simulink library "carnot"  (R2013b)
settings: Solver=ode45  StartTime=0.0  StopTime=10.0  RelTol=1e-3
undefined symbols (not defined in the file or in its folder): A, acol, Ahabit, Awin, Azimuth_Angle, AziWin, B, C, c1, c4, capc, caph, CarnotCallbacks_Density, CarnotCallbacks_Enthalpy, CarnotCallbacks_Enthalpy2Temperature, CarnotCallbacks_Entropy, CarnotCallbacks_Evaporation_Enthalpy, CarnotCallbacks_GlobalMessageLevel, CarnotCallbacks_Grashof, CarnotCallbacks_Heat_Capacity, CarnotCallbacks_Kinematic_Viscosity, CarnotCallbacks_Prandtl, CarnotCallbacks_Saturation_Property, CarnotCallbacks_Saturation_Temperature, CarnotCallbacks_Saturation_Value_Water, CarnotCallbacks_Specific_Volume, CarnotCallbacks_Thermal_Conductivity, CarnotCallbacks_Vapour_Content, CarnotCallbacks_Vapour_Pressure, con, cond, d, Dd, density, dfin, dia, DiameterLastPiece, DPConstant, dpipe, DPLinear, DPQuadratic, emission_out, fluid, FluidMix, FluidType, FPC, frame, g, GeodeticHeight, Gwin, heat_capacity, hgt, HP, Hroom, ID, inlet, K, l, lin, lpipe ... (+29)
undefined symbols (not defined in the file): c2, c3, c5, c6, cwall, dactive, height, mc, mID, rho, tau, UAneighbour, UAwall, uloss
libraries: carnot x333, simulink x25, simulink_extras x7
(part 14 of 16)

== system carnot/Load/Houses/room_nodes/Room_Node ==
  note: r: radiative
      | c: convective
  note: NODE of a ZONE ( heat flow, temperature, ventilation / infiltration and energy consumption)
  sum([S]) : Inport
  1/s to 1/h : Gain  Gain=3600  SaturateOnIntegerOverflow=on  OutDataTypeStr=Inherit: Same as input  ParamDataTypeStr=Inherit: Same as input
  Demux2 : Demux  Outputs=13
  Mux2 : Mux  Inputs=6
  Mux3 : Mux  Inputs=9
  Sensitive room temperature : Subsystem  mask(SENSITIVE TEMPERATURE){share_c=47}
      mask prompts: share_c "SHARE of convective sensitivity, [0,100%]:"
      mask help:
      | This block merges the convective and radiative zone node temperature to the SENSITIVE ZONE TEMPERATURE (weighted arithmetic average of both components).
      |
      | [T] = [Tc; Tr]:  temperature vector of node, °C
      | Ts:              sensitive zone temperature, °C
      mask init: same as carnot/Outputs/Sensitive_Room_Temperature
  Terminator : Terminator
  convective_node : Subsystem
  m^3 : Constant  Value=zoneairvolume
  radiative_node : Subsystem
  "[AIV]" : Outport
  "[S]" : Outport  Port=2
  Qdot_sol : Outport  Port=3
  Vair : Outport  Port=4
  wires:
  m^3/1 -> Vair/1
  Mux2/1 -> Terminator/1  "[Qdot]"
  sum([S])/1 -> "[S]"/1, Demux2/1
  Demux2/8 -> radiative_node/1(Qdotr)  "Qdotr"
  Demux2/7 -> convective_node/1(Qdotc)  "Qdotc"
  Demux2/6 -> Mux2/6  "Qdot_air"
  Demux2/5 -> Mux2/5  "Qdot_heat"
  Demux2/4 -> Mux2/4  "Qdot_pers"
  Demux2/3 -> Mux2/3  "Qdot_light"
  Demux2/2 -> Mux2/2  "Qdot_equip"
  Demux2/1 -> Mux2/1, Qdot_sol/1  "Qdot_sol"
  1/s to 1/h/1 -> Mux3/9  "nair_out"
  convective_node/2(x_H2O) -> Mux3/4  "x_H2O"
  convective_node/3(x_CO2) -> Mux3/5  "x_CO2"
  convective_node/6(p) -> Mux3/8  "p"
  convective_node/5(cp) -> Mux3/7  "cp"
  convective_node/4(rho) -> Mux3/6  "rho"
  convective_node/7(nair_out) -> 1/s to 1/h/1
  convective_node/1(Tc) -> Sensitive room temperature/2(Tc), Mux3/2  "Tc"
  radiative_node/1(Tr) -> Sensitive room temperature/1(Tr), Mux3/3  "Tr"
  Demux2/9 -> convective_node/2(mdot_air)  "mdot_air"
  Demux2/10 -> convective_node/3(mdot_H2O)  "mdot_H2O"
  Demux2/11 -> convective_node/4(mdot_CO2)  "mdot_CO2"
  Demux2/12 -> convective_node/5(Vdot_out2in)  "Vdot_out2in"
  Demux2/13 -> convective_node/6(Vdot_in2out)  "Vdot_in2out"
  Mux3/1 -> "[AIV]"/1
  Sensitive room temperature/1(Ts) -> Mux3/1  "Ts"

== system carnot/Load/Houses/ventilation_heating/Floorheating_TABS ==
  note: source: Koschenz, M.; Lehmann, B.: Thermoaktive Bauteilsysteme tabs. EMPA, Dübendorf, 2000. ISBN 3-905594-19-6
  T(P) : Inport
  THBin : Inport  Port=2
  Bus Assignment : BusAssignment  AssignedSignals=Temperature
  Bus Selector : BusSelector  OutputSignals=Temperature,MassFlow,Pressure,FluidType,FluidMix
  Demux2 : Demux  Outputs=2
  Mux2 : Mux  Inputs=6
  S-Function : S-Function  FunctionName=tabs  Parameters=d d1 d_pipe dr dx l lambda_r lambda_b  EnableBusSupport=off
  power : Outport
  THBout : Outport  Port=2  InitialOutput=0
  wires:
  T(P)/1 -> Mux2/6
  THBin/1 -> Bus Assignment/1, Bus Selector/1
  Bus Selector/4 -> Mux2/4  "<FluidType>"
  Bus Selector/3 -> Mux2/3  "<Pressure>"
  Bus Selector/2 -> Mux2/2  "<MassFlow>"
  Bus Selector/5 -> Mux2/5  "<FluidMix>"
  Bus Selector/1 -> Mux2/1  "<Temperature>"
  Mux2/1 -> S-Function/1
  S-Function/1 -> Demux2/1
  Demux2/2 -> Bus Assignment/2  "Temperature"
  Demux2/1 -> power/1
  Bus Assignment/1 -> THBout/1

== system carnot/Load/Houses/ventilation_heating/THB_P_adapter ==
  note: (°C)
  T(P) : Inport
  THBin : Inport  Port=2
  -1 : Gain  Gain=-1  SaturateOnIntegerOverflow=on  OutDataTypeStr=Inherit: Same as input  ParamDataTypeStr=Inherit: Same as input
  Bus Assignment : BusAssignment  AssignedSignals=Temperature
  Bus Selector : BusSelector  OutputSignals=Temperature,MassFlow
  Heat_Capacity : carnot/Basic/Material_Properties/Heat_Capacity  VariantControl=CarlibClassic  INPUTARGUMENTS=THB  DEBUGLEVEL=DEBUGLEVEL  MAXTOTALWARNINGS=inf  MAXCONSECUTIVEWARNINGS=inf  WRITETOFILE=0  FILENAME='errors.txt'
  Integrator : Integrator  InitialCondition=t0
  Product1 : Product  Inputs=3  SaturateOnIntegerOverflow=on  InputSameDT=on  OutDataTypeStr=Inherit: Same as first input
  Product2 : Product  Inputs=/*  SaturateOnIntegerOverflow=on  InputSameDT=on  OutDataTypeStr=Inherit: Same as first input
  Sum1 : Sum  Inputs=-+  SaturateOnIntegerOverflow=on  InputSameDT=on  OutDataTypeStr=Inherit: Same as first input
  Sum2 : Sum  SaturateOnIntegerOverflow=on  InputSameDT=on  OutDataTypeStr=Inherit: Same as first input
  Sum3 : Sum  Inputs=+-  SaturateOnIntegerOverflow=on  InputSameDT=on  OutDataTypeStr=Inherit: Same as first input
  heat transfer : Gain  Gain=ua  SaturateOnIntegerOverflow=on  OutDataTypeStr=Inherit: Same as input  ParamDataTypeStr=Inherit: Same as input
  mass : Gain  Gain=mass  SaturateOnIntegerOverflow=on  OutDataTypeStr=Inherit: Same as input  ParamDataTypeStr=Inherit: Same as input
  power : Outport  InitialOutput=0
  THB : Outport  Port=2  InitialOutput=0
  wires:
  Bus Assignment/1 -> THB/1
  Sum3/1 -> Product1/1
  Bus Selector/2 -> Product1/2  "<MassFlow>"
  Product1/1 -> Sum2/1
  Heat_Capacity/1 -> Product1/3, mass/1
  Bus Selector/1 -> Sum3/1  "<Temperature>"
  Sum1/1 -> heat transfer/1
  T(P)/1 -> Sum1/2  "Tnode"
  Integrator/1 -> Sum1/1, Bus Assignment/2, Sum3/2  "Twater"
  mass/1 -> Product2/1
  Product2/1 -> Integrator/1
  Sum2/1 -> Product2/2
  -1/1 -> power/1
  heat transfer/1 -> Sum2/2, -1/1  "Qdot"
  THBin/1 -> Heat_Capacity/1, Bus Assignment/1, Bus Selector/1

== system carnot/Load/Houses/wall_floor/Floor_in ==
  "[AIV]floor" : Inport
  power per node : Inport  Port=2
  "[AIV]ceiling" : Inport  Port=3
  Qdot_sol : Inport  Port=4
  Mux : Mux  Inputs=3
  Wall_basic : carnot/Basic/Thermal_Models/Wall_basic  tau=tau  t0=t0  d=d  dactive=dactive  cond=cond  cwall=cwall  rho=rho
  alfa_ceiling : carnot/Load/Houses/heat_transfer/alfa_ceiling  active=active  emission_c=emission_c  wallsurface=wallsurface
  alfa_floor : carnot/Load/Houses/heat_transfer/alfa_floor  active=active  emission_f=emission_f  wallsurface=wallsurface
  per surface : Gain  Gain=1/wallsurface  SaturateOnIntegerOverflow=on  OutDataTypeStr=Inherit: Same as input  ParamDataTypeStr=Inherit: Same as input
  "[S]floor" : Outport
  T(P) : Outport  Port=2
  "[S]ceiling" : Outport  Port=3
  Tn : Outport  Port=4
  wires:
  Wall_basic/2 -> Mux/2, T(P)/1
  "[AIV]ceiling"/1 -> alfa_ceiling/2
  alfa_ceiling/2 -> "[S]ceiling"/1
  alfa_floor/2 -> "[S]floor"/1
  "[AIV]floor"/1 -> alfa_floor/2
  Wall_basic/3 -> Mux/3, alfa_ceiling/1
  Wall_basic/1 -> Mux/1, alfa_floor/1
  alfa_floor/1 -> Wall_basic/1
  alfa_ceiling/1 -> Wall_basic/3
  Qdot_sol/1 -> alfa_floor/3
  power per node/1 -> per surface/1
  per surface/1 -> Wall_basic/2
  Mux/1 -> Tn/1

== system carnot/Load/Houses/wall_floor/Roof ==
  WDB : Inport
  power per node : Inport  Port=2
  "[AIV]" : Inport  Port=3
  Mux : Mux  Inputs=3
  Wall_basic : carnot/Basic/Thermal_Models/Wall_basic  tau=tau  t0=t0  d=d  dactive=dactive  cond=cond  cwall=cwall  rho=rho
  alfa_ceiling : carnot/Load/Houses/heat_transfer/alfa_ceiling  active=active  emission_c=emission_c  wallsurface=wallsurface
  alfa_wall_out : carnot/Load/Houses/heat_transfer/alfa_wall_out  pos=0  absorption_out=0.4  emission_out=0.7  wallsurface=1
  per surface : Gain  Gain=1/wallsurface  SaturateOnIntegerOverflow=on  OutDataTypeStr=Inherit: Same as input  ParamDataTypeStr=Inherit: Same as input
  "[S]" : Outport
  Tn : Outport  Port=2
  wires:
  per surface/1 -> Wall_basic/2
  power per node/1 -> per surface/1
  alfa_ceiling/2 -> "[S]"/1
  "[AIV]"/1 -> alfa_ceiling/2
  alfa_ceiling/1 -> Wall_basic/3
  Wall_basic/2 -> Mux/2
  Wall_basic/3 -> Mux/3, alfa_ceiling/1
  Wall_basic/1 -> Mux/1, alfa_wall_out/2
  WDB/1 -> alfa_wall_out/1
  alfa_wall_out/1 -> Wall_basic/1
  Mux/1 -> Tn/1

== system carnot/Load/Houses/wall_floor/Wall_in ==
  "[AIV]" : Inport
  power per node : Inport  Port=2
  "[AIV]n" : Inport  Port=3
  Mux : Mux  Inputs=3
  Wall_basic : carnot/Basic/Thermal_Models/Wall_basic  tau=tau  t0=t0  d=d  dactive=dactive  cond=cond  cwall=cwall  rho=rho
  alfa_wall_in : carnot/Load/Houses/heat_transfer/alfa_wall_in  active=active  emission_in=emission_in  wallsurface=wallsurface
  alfa_wall_in1 : carnot/Load/Houses/heat_transfer/alfa_wall_in  active=active  emission_in=emission_in  wallsurface=wallsurface
  per surface : Gain  Gain=1/wallsurface  SaturateOnIntegerOverflow=on  OutDataTypeStr=Inherit: Same as input  ParamDataTypeStr=Inherit: Same as input
  "[S]" : Outport
  "[S]n" : Outport  Port=2
  Tn : Outport  Port=3
  wires:
  Mux/1 -> Tn/1
  Wall_basic/2 -> Mux/2
  alfa_wall_in1/2 -> "[S]n"/1
  "[AIV]n"/1 -> alfa_wall_in1/2
  Wall_basic/3 -> alfa_wall_in1/1, Mux/3
  alfa_wall_in1/1 -> Wall_basic/3
  "[AIV]"/1 -> alfa_wall_in/2
  Wall_basic/1 -> Mux/1, alfa_wall_in/1
  alfa_wall_in/2 -> "[S]"/1
  alfa_wall_in/1 -> Wall_basic/1
  per surface/1 -> Wall_basic/2
  power per node/1 -> per surface/1

== system carnot/Load/Houses/wall_floor/Wall_out ==
  WDB : Inport
  power per node : Inport  Port=2
  "[AIV]" : Inport  Port=3
  Mux : Mux  Inputs=3
  Wall_basic : carnot/Basic/Thermal_Models/Wall_basic  tau=tau  t0=t0  d=d  dactive=dactive  cond=cond  cwall=cwall  rho=rho
  alfa_wall_in : carnot/Load/Houses/heat_transfer/alfa_wall_in  active=active  emission_in=emission_in  wallsurface=wallsurface
  alfa_wall_out : carnot/Load/Houses/heat_transfer/alfa_wall_out  pos=pos  absorption_out=absorption_out  emission_out=emission_out  wallsurface=wallsurface
  per surface : Gain  Gain=1/wallsurface  SaturateOnIntegerOverflow=on  OutDataTypeStr=Inherit: Same as input  ParamDataTypeStr=Inherit: Same as input
  "[S]" : Outport
  Tn : Outport  Port=2
  wires:
  alfa_wall_in/2 -> "[S]"/1
  "[AIV]"/1 -> alfa_wall_in/2
  Wall_basic/3 -> Mux/3, alfa_wall_in/1
  alfa_wall_in/1 -> Wall_basic/3
  Wall_basic/1 -> Mux/1, alfa_wall_out/2
  alfa_wall_out/1 -> Wall_basic/1
  per surface/1 -> Wall_basic/2
  power per node/1 -> per surface/1
  WDB/1 -> alfa_wall_out/1
  Wall_basic/2 -> Mux/2
  Mux/1 -> Tn/1

== system carnot/Load/Houses/wall_floor/Wall_with_Window ==
  WDB : Inport
  "[AIV]" : Inport  Port=2
  Ground : Ground
  Wall_out : carnot/Load/Houses/wall_floor/Wall_out  wallsize=[wallsize windowsize]  pos=pos  t0=t0  d=[0.1 0.38]  cond=[0.04 0.79]  cwall=[0.28 0.28]*3600  rho=[900 1800]  reflectground=0.3  abs_emiss=[0.65 0.97 0.96]  tau=tau  dactive=-1
  Window : carnot/Load/Houses/wall_floor/Window  wallsize=windowsize  frame=frame  pos=pos  t0=t0  d=[0.03 0.03]  cond=[.81 .81]  cwall=[.28 .28]*3600  rho=[2500 2500]  misc=[0.2 0.1 1 1]  gvalue=g  tau=tau  dactive=[0.01 0.05]
  "[S]wall" : Outport
  "[S]window" : Outport  Port=2
  wires:
  Window/1 -> "[S]window"/1
  Wall_out/1 -> "[S]wall"/1
  Ground/1 -> Wall_out/2
  "[AIV]"/1 -> Window/2, Wall_out/3
  WDB/1 -> Window/1, Wall_out/1

== system carnot/Load/Houses/wall_floor/Window ==
  WDB : Inport
  "[AIV]" : Inport  Port=2
  Terminator1 : Terminator
  Wall_basic : carnot/Basic/Thermal_Models/Wall_basic  tau=tau  t0=t0  d=d  dactive=dactive  cond=cond  cwall=cwall  rho=rho
  alfa_window_in : carnot/Load/Houses/heat_transfer/alfa_window_in  gvalue=0.7  emission_in=0.87  wallsurface=1  frame=0.1  numlayer=2
  alfa_window_out : carnot/Load/Houses/heat_transfer/alfa_window_out  pos=0  absorption_out=0.01  emission_out=0.87  frame=0.1
  position1 : Constant  Value=gvalue
  "[S]" : Outport
  wires:
  Wall_basic/1 -> alfa_window_out/3
  position1/1 -> alfa_window_out/2
  "[AIV]"/1 -> alfa_window_in/3
  alfa_window_in/1 -> Wall_basic/3
  alfa_window_in/3 -> "[S]"/1
  WDB/1 -> alfa_window_out/1
  alfa_window_out/1 -> alfa_window_in/2
  Wall_basic/2 -> Terminator1/1
  alfa_window_out/2 -> Wall_basic/1
  Wall_basic/3 -> alfa_window_in/1
  alfa_window_in/2 -> Wall_basic/2

== system carnot/Load/Houses/wall_floor/Window_Optics ==
  WDB : Inport
  Bus Selector : BusSelector  OutputSignals=Incidence_Angle_sun,Solar_Radiation_direct_surface,Solar_Radiation_diffuse_surface
  IAM diffuse : Gain  Gain=0.8  SaturateOnIntegerOverflow=on  OutDataTypeStr=Inherit: Same as input  ParamDataTypeStr=Inherit: Same as input
  IAM window : Lookup  InputValues=[-10 0 50 70 80 90]  Table="[1.0 1.0  0.95  0.7  0.0  0.0]"  SaturateOnIntegerOverflow=on
  Product : Product
  Sum : Sum  SaturateOnIntegerOverflow=on  InputSameDT=on  OutDataTypeStr=Inherit: Same as first input
  qsolar : Outport
  wires:
  Bus Selector/3 -> IAM diffuse/1  "<Solar_Radiation_diffuse_surface>"
  IAM window/1 -> Product/1
  IAM diffuse/1 -> Sum/2
  Product/1 -> Sum/1
  Sum/1 -> qsolar/1
  Bus Selector/1 -> IAM window/1  "<Incidence_Angle_sun>"
  Bus Selector/2 -> Product/2  "<Solar_Radiation_direct_surface>"
  WDB/1 -> Bus Selector/1

== system carnot/Load/Houses/wall_floor/Window_with_Shading ==
  WDB : Inport
  "[AIV]" : Inport  Port=2
  control : Inport  Port=3
  alfa_window_in : Subsystem  mask(ALFA){}
      mask help:
      | Convective and radiative heat transfer at the INDOOR SURFACE OF A VERTICAL WINDOW with 1-4 layers (each 3 ... 8 mm thick).
      |
      | Ts  : temperature of window surface, °C,
      | [sun_t]  : sun data (incidence angle, direct and diffuse radiation
      |     at tilted window surface),
      | [AIV]  : conditions of zone node,
      | qdots  : specific heat flow into window construction, W/m^2,
      | [S]  : heat and air flow to zone node.
  alfa_window_out : carnot/Load/Houses/heat_transfer/alfa_window_out  pos=0  absorption_out=0.01  emission_out=0.87  frame=0.1
  lambda_window : Subsystem  mask(LAMBDA){}
      mask help:
      | Heat conduction through a transparent component (window).
      |
      | qdots1	: specific heat flow vertical on surface 1, W/m²
      | qdots2	: specific heat flow vertical on surface 2, W/m²
      | Ts1	: temperature of surface 1, °C
      | Ts2	: temperature of surface 2, °C
      |
      | NOTE CONVENTION for INPUT NUMBER:
      | "1"	  indoor surface of an outer window OR
      | 	  surface "a" of an inner window OR
      |  	  surface "f" of a glass floor
      |
      | "2"	  outdoor surface of a window OR
      | 	  surface "b" of an inner window OR
      |  	  surface "c" of a glass ceiling
  position1 : Constant  Value=gvalue
  "[S]" : Outport
  wires:
  lambda_window/1(Ts1) -> alfa_window_out/3
  WDB/1 -> alfa_window_in/4(WDB), alfa_window_out/1
  "[AIV]"/1 -> alfa_window_in/3("[AIV]")
  alfa_window_in/1(qdots2) -> lambda_window/2(qdots2)
  alfa_window_in/2("[S]") -> "[S]"/1
  lambda_window/2(Ts2) -> alfa_window_in/1(Ts2)
  alfa_window_out/2 -> lambda_window/1(qdots1)
  alfa_window_out/1 -> alfa_window_in/2("[sun_t]")
  control/1 -> alfa_window_in/5(control)
  position1/1 -> alfa_window_out/2

== system carnot/Source/Chiller/Absorption_Chiller_ddT/Transfer Fcn (with initial states) ==
  In1 : Inport
  State Space : StateSpace  A=A  B=B  C=C  D=Dd  X0=X0
  Out1 : Outport  InitialOutput=0
  wires:
  In1/1 -> State Space/1
  State Space/1 -> Out1/1

== system carnot/Source/Chiller/Absorption_Chiller_ddT/absorber // condenser ==
  note: Qdot_E + Qdot_G = Qdot_A + Qdot_C
  THBcooler_in : Inport
  Qdot_E_act [W] : Inport  Port=2
  Qdot_G [W] : Inport  Port=3
  on : Inport  Port=4
  Add1 : Sum
  Bus Assignment : BusAssignment  AssignedSignals=Temperature
  Bus Selector : BusSelector  OutputSignals=Temperature,MassFlow,Pressure,FluidType,FluidMix
  Tcooler_out : Subsystem
  prod : Product
  THBcooler : Outport
  t_AC : Outport  Port=2
  wires:
  Tcooler_out/1(Tcooler_out) -> Bus Assignment/2
  Bus Assignment/1 -> THBcooler/1
  prod/1 -> Tcooler_out/3(Qdot_E + Qdot_G)
  Add1/1 -> prod/2
  on/1 -> prod/1
  Qdot_G [W]/1 -> Add1/2
  Qdot_E_act [W]/1 -> Add1/1
  THBcooler_in/1 -> Bus Assignment/1, Bus Selector/1
  Bus Selector/5 -> Tcooler_out/6(mix)  "<FluidMix>"
  Bus Selector/4 -> Tcooler_out/5(fluid)  "<FluidType>"
  Bus Selector/3 -> Tcooler_out/4(p)  "<Pressure>"
  Bus Selector/1 -> t_AC/1, Tcooler_out/1(T)  "<Temperature>"
  Bus Selector/2 -> Tcooler_out/2(mdot)  "<MassFlow>"

== system carnot/Source/Chiller/Absorption_Chiller_ddT/boiler ==
  THBhot_in : Inport
  deltadelta_t : Inport  Port=2
  on : Inport  Port=3
  Bus Assignment : BusAssignment  AssignedSignals=Temperature
  Bus Selector : BusSelector  OutputSignals=Temperature,MassFlow,Pressure,FluidType,FluidMix
  Pressure_Drop_Fix : carnot/Basic/Pressure_Drop/Pressure_Drop_Fix  con=0  lin=dpg(1)  qua=dpg(2)
  Qdot_G with deltadelta_t : Subsystem
  Thot_out : Subsystem
  prod : Product
  THVhot_out : Outport
  t_B : Outport  Port=2
  Qdot_G [W] : Outport  Port=3
  wires:
  Pressure_Drop_Fix/1 -> THVhot_out/1
  Thot_out/1(Thot_out) -> Bus Assignment/2
  Bus Assignment/1 -> Pressure_Drop_Fix/1
  THBhot_in/1 -> Bus Assignment/1, Bus Selector/1
  Qdot_G with deltadelta_t/1(Qdot_G [W]) -> prod/2
  on/1 -> prod/1
  prod/1 -> Qdot_G [W]/1, Thot_out/3(Qdot_G)
  deltadelta_t/1 -> Qdot_G with deltadelta_t/1(deltadelta_t)
  Bus Selector/5 -> Thot_out/6(mix)  "<FluidMix>"
  Bus Selector/4 -> Thot_out/5(fluid)  "<FluidType>"
  Bus Selector/3 -> Thot_out/4(p)  "<Pressure>"
  Bus Selector/1 -> t_B/1, Thot_out/1(Thot_in)  "<Temperature>"
  Bus Selector/2 -> Thot_out/2(mdot)  "<MassFlow>"

== system carnot/Source/Chiller/Absorption_Chiller_ddT/deltadelta_t ==
  note: deltadelta_t = t_B - (1+E) * t_AC + E * t_E
  t_B : Inport
  t_E : Inport  Port=2
  t_AC : Inport  Port=3
  Add : Sum  Inputs=++-
  Gain : Gain  Gain=1+E
  Gain1 : Gain  Gain=E
  deltadelta_t : Outport
  wires:
  t_AC/1 -> Gain/1
  t_E/1 -> Gain1/1
  Add/1 -> deltadelta_t/1
  t_B/1 -> Add/1
  Gain1/1 -> Add/2
  Gain/1 -> Add/3

== system carnot/Source/Chiller/Absorption_Chiller_ddT/evaporator ==
  THBload_in : Inport
  deltadelta_t : Inport  Port=2
  on : Inport  Port=3
  Bus Assignment : BusAssignment  AssignedSignals=Temperature
  Bus Selector : BusSelector  OutputSignals=Temperature,MassFlow,Pressure,FluidType,FluidMix
  Pressure_Drop_Fix : carnot/Basic/Pressure_Drop/Pressure_Drop_Fix  con=0  lin=dpe(1)  qua=dpe(2)
  Qdot_E with deltadelta_t : Subsystem
  Tchilled_out : Subsystem
  prod : Product
  THBload : Outport
  t_E : Outport  Port=2
  Qdot_E [W] : Outport  Port=3
  wires:
  Pressure_Drop_Fix/1 -> THBload/1
  Bus Assignment/1 -> Pressure_Drop_Fix/1
  THBload_in/1 -> Bus Assignment/1, Bus Selector/1
  Qdot_E with deltadelta_t/1(Qdot_E [W]) -> prod/2
  prod/1 -> Qdot_E [W]/1, Tchilled_out/3(Qdot_E)
  on/1 -> prod/1
  Bus Selector/3 -> Tchilled_out/4(p)  "<Pressure>"
  Tchilled_out/1(Tcold) -> Bus Assignment/2, t_E/1
  deltadelta_t/1 -> Qdot_E with deltadelta_t/1(deltadelta_t)
  Bus Selector/5 -> Tchilled_out/6(mix)  "<FluidMix>"
  Bus Selector/4 -> Tchilled_out/5(fluid)  "<FluidType>"
  Bus Selector/1 -> Tchilled_out/1(T)  "<Temperature>"
  Bus Selector/2 -> Tchilled_out/2(mdot)  "<MassFlow>"

== system carnot/Source/Chiller/Compression_Air_Water_Chiller/Lookup_tables _COP + Q_cold_faktor ==
  T_AIR_IN : Inport
  T_WATER_OUT : Inport  Port=2
  control_AC : Inport  Port=3
  Constant : Constant  Value=Q_Nom
  Gain : Gain  Gain=1000
  Product : Product  RndMeth=Zero
  Product1 : Product  Inputs=4  RndMeth=Zero
  Product2 : Product  Inputs=/*  RndMeth=Zero
  lookup_table_COP : Lookup_n-D  BreakpointsForDimension1=[7,18]  BreakpointsForDimension2=[15,20,25,30,35,40]  BreakpointsForDimension3=[1:2]  BreakpointsForDimension4=[1:2]  Table=[3.55 3.15 2.65 2.25 2 1.7;3.8 3.4 2.93 2.58 2.2 1.95]  InputSameDT=on
  lookup_table_Q_cold_faktor : Lookup_n-D  BreakpointsForDimension1=[7,18]  BreakpointsForDimension2=[15,20,25,30,35,40]  BreakpointsForDimension3=[1:2]  BreakpointsForDimension4=[1:2]  Table=|  InputSameDT=on
      | [ 1.26 1.19 1.08 1.00 0.90 0.79;
      |              1.65 1.53 1.41 1.28 1.18 1.09]
  runtime_AC : Subsystem  TreatAsAtomicUnit=on
      mask help: This block counts the time if input is set to one, it stops counting if input is zero and continues when input rises to one again.
      mask Help: eval('filetest (''manual.htm#count_working_time'')')
  start-up-faktor : Fcn  Expr=1-exp(-u/(150/5))
  COP : Outport
  Q_cold : Outport  Port=2
  P_el : Outport  Port=3
  wires:
  Gain/1 -> Q_cold/1, Product2/2
  T_WATER_OUT/1 -> lookup_table_Q_cold_faktor/1, lookup_table_COP/1
  T_AIR_IN/1 -> lookup_table_Q_cold_faktor/2, lookup_table_COP/2
  lookup_table_COP/1 -> Product/1, Product2/1
  control_AC/1 -> Product/2, runtime_AC/1(control_AC), Product1/2
  lookup_table_Q_cold_faktor/1 -> Product1/3
  runtime_AC/1(runtime) -> start-up-faktor/1
  Product/1 -> COP/1
  Product1/1 -> Gain/1
  start-up-faktor/1 -> Product1/1
  Constant/1 -> Product1/4
  Product2/1 -> P_el/1

== system carnot/Source/Chiller/Compression_Air_Water_Chiller/cooling ==
  THB_in : Inport
  Q_cold : Inport  Port=2
  Bus Assignment : BusAssignment  AssignedSignals=Temperature
  Bus Selector : BusSelector  OutputSignals=Temperature,MassFlow
  Constant : Constant  Value=20
  Constant_THB : carnot/Source/Simple/Constant_THB  t=40  mdot=0*100/3600  p=1e5  mID=No Pressure Drop  fluid=Water  mix=0  dia=0.02  hgt=0
  Heat_Capacity : carnot/Basic/Material_Properties/Heat_Capacity  VariantControl=CarlibClassic  INPUTARGUMENTS=THB  DEBUGLEVEL=DEBUGLEVEL  MAXTOTALWARNINGS=inf  MAXCONSECUTIVEWARNINGS=inf  WRITETOFILE=0  FILENAME='errors.txt'
  Product : Product  Inputs=//*  SaturateOnIntegerOverflow=on  RndMeth=Zero  InputSameDT=on  OutDataTypeStr=Inherit: Same as first input
  Saturation : Saturate  UpperLimit=inf  LowerLimit=1
  Storage_Type_1 : carnot/Storage/Thermal/Storage_Type_1  uloss=1  ubot=1  utop=1  cond=1  t0=[10:5:55]  volume=0.03  dia=0.01  pos=standing cylinder  nconnect=2  nodes=10  mpoints=10
  Sum2 : Sum  Inputs=+-  InputSameDT=on  OutDataTypeStr=Inherit: Same as first input
  Terminator : Terminator
  Terminator1 : Terminator
  Terminator2 : Terminator
  isinf : MATLAB Function  TreatAsAtomicUnit=on
  isnan : MATLAB Function  TreatAsAtomicUnit=on
  THB_out : Outport
  wires:
  Storage_Type_1/3 -> Terminator2/1
  Storage_Type_1/2 -> Terminator1/1
  Storage_Type_1/1 -> Terminator/1
  Storage_Type_1/4 -> THB_out/1
  Bus Selector/2 -> Product/1  "<MassFlow>"
  Heat_Capacity/1 -> Product/2
  Bus Assignment/1 -> Storage_Type_1/3
  Constant/1 -> Storage_Type_1/1
  Constant_THB/1 -> Storage_Type_1/2
  THB_in/1 -> Heat_Capacity/1, Bus Selector/1, Bus Assignment/1
  Bus Selector/1 -> Sum2/1  "<Temperature>"
  Q_cold/1 -> Product/3  "W"
  isnan/1(y) -> isinf/1(u)
  Product/1 -> isnan/1(u)
  isinf/1(y) -> Sum2/2
  Sum2/1 -> Saturation/1
  Saturation/1 -> Bus Assignment/2

== system carnot/Source/Chiller/Compression_Air_Water_Chiller/measure_T_WATER_OUT ==
  THV_in : Inport
  Demux3 : Demux  Outputs=2
  Terminator : Terminator
  heat capacity : StateSpace  A=-tc  B=tc  D=0  X0=t0
  select temperature : Selector  InputPortWidth=5  IndexOptions=Index vector (dialog)  Indices=[2]  OutputSizes=1
  T : Outport
  THV : Outport  Port=2
  wires:
  Demux3/2 -> Terminator/1
  Demux3/1 -> select temperature/1
  THV_in/1 -> Demux3/1, THV/1
  select temperature/1 -> heat capacity/1
  heat capacity/1 -> T/1

== system carnot/Source/Chiller/Cooling_Tower/Fan ==
  note: Grundlage zur Berechnung
      | bei Drehzahländerung eines bestimmten Lüfters
      |
      | Proportionalitätsgesetz
      | V1/V2 = n1/n2
      | P1/P2 = (n1/n2)^3
      |
      | Wirkungsgrad Elektromotor
      | P = Pm/eta
  n_fan : Inport
  Divide1 : Product  Inputs=*/
  Divide2 : Product  Inputs=*/*
  Divide3 : Product  Inputs=/*
  Divide4 : Product  Inputs=/*
  Input Leistung : Constant  Value=1.8
  Math Function : Math  Operator=pow  SaturateOnIntegerOverflow=on
  Pw1 : Constant  Value=3
  max. Drehzahl : Constant  Value=824
  max. Vdot_Lüfter : Constant  Value=2.2
  n_fan [%] : Outport
  vdot_fan : Outport  Port=2
  P_fan : Outport  Port=3
  wires:
  n_fan/1 -> Divide2/1, Divide4/1, Divide1/1
  max. Drehzahl/1 -> Divide2/2, Divide1/2, Divide4/2
  Divide1/1 -> n_fan [%]/1
  Input Leistung/1 -> Divide3/2
  max. Vdot_Lüfter/1 -> Divide2/3
  Divide2/1 -> vdot_fan/1
  Divide3/1 -> P_fan/1
  Divide4/1 -> Math Function/1
  Math Function/1 -> Divide3/1
  Pw1/1 -> Math Function/2

== system carnot/Source/Chiller/Cooling_Tower/Feuchtkugel- temperatureinfluss // wet-bulb temperature effect ==
  WDB : Inport
  t_ie : Inport  Port=2
  Enable : EnablePort
  "Abgleich " : Subsystem
  Add : Sum
  Constant : Constant  Value=2
  Divide : Product  Inputs=*/
  THB_WetBulbTemperature : carnot/Basic/Material_Properties/THB_WetBulbTemperature
  Terminator1 : Terminator
  WDB2THB : carnot/Weather/WDB2THB  dia=0.2
  wet-bulb 15 °C : Subsystem
  t_FK : Outport  InitialOutput=0
  t_ia_FK : Outport  Port=2  InitialOutput=0
  dt : Outport  Port=3  InitialOutput=0
  wires:
  WDB2THB/1 -> THB_WetBulbTemperature/1
  THB_WetBulbTemperature/2 -> Terminator1/1
  WDB/1 -> WDB2THB/1
  wet-bulb 15 °C/1(t_ia_FK15) -> "Abgleich "/3(t_ia_FK15)
  THB_WetBulbTemperature/1 -> "Abgleich "/1(t_FK), t_FK/1
  t_ie/1 -> Add/2, wet-bulb 15 °C/1(t_ie), "Abgleich "/2(t_ie)
  "Abgleich "/1(t_ia_FK) -> Add/1, t_ia_FK/1
  Add/1 -> Divide/1
  Constant/1 -> Divide/2
  Divide/1 -> dt/1

== system carnot/Source/Chiller/Cooling_Tower/Leistungseinflüsse // influence on coolingpower ==
  t_ia_FK : Inport
  cp_i : Inport  Port=2
  t_ie : Inport  Port=3
  mdot_i : Inport  Port=4
  Fluid_Type : Inport  Port=5
  Fluid_mix : Inport  Port=6
  n_fan [%] : Inport  Port=7
  Enable : EnablePort
  Qdot_i_FK : Subsystem
  "Qdot_i_ist " : Subsystem
  "t_ia_ist " : Subsystem
  Qdot_i_ist : Outport  InitialOutput=0
  t_ia_ist : Outport  Port=2  InitialOutput=0
  wires:
  "Qdot_i_ist "/1(Qdot_i_ist) -> Qdot_i_ist/1, "t_ia_ist "/1(Qdot_i_ist)
  Qdot_i_FK/1(Qdot_i_FK) -> "Qdot_i_ist "/1(Qdot_i_FK)
  t_ie/1 -> Qdot_i_FK/2(t_ie), "t_ia_ist "/2(t_ie), "Qdot_i_ist "/6(t_ie)
  t_ia_FK/1 -> Qdot_i_FK/1(t_ia_FK)
  n_fan [%]/1 -> "Qdot_i_ist "/2(n_Fan [%])
  "t_ia_ist "/1(t_ia_ist) -> t_ia_ist/1
  cp_i/1 -> "t_ia_ist "/3(cp_i)
  Fluid_Type/1 -> Qdot_i_FK/3(Fluid_Type), "Qdot_i_ist "/5(Fluid_Type)
  mdot_i/1 -> "Qdot_i_ist "/4(mdot_i), "t_ia_ist "/4(mdot)
  Fluid_mix/1 -> "Qdot_i_ist "/3(Fluid_mix)

== system carnot/Source/Chiller/Cooling_Tower/Verbrauch // consumption ==
  Qdot : Inport
  vdot_fan : Inport  Port=2
  P_fan : Inport  Port=3
  control_fan : Inport  Port=4
  phi_le : Inport  Port=5
  t_le : Inport  Port=6
  t_ie : Inport  Port=7
  Strom : Subsystem
  Verdunstung : Subsystem
  energy : Outport
  power : Outport  Port=2
  Wasserverbrauch : Outport  Port=3
  wires:
  control_fan/1 -> Strom/1(control_Fan), Verdunstung/1(control_Fan)
  P_fan/1 -> Strom/2(P_Fan)
  Strom/2(power) -> power/1
  t_le/1 -> Verdunstung/2(t_le)
  Verdunstung/1(Wasserverbrauch) -> Wasserverbrauch/1
  phi_le/1 -> Verdunstung/3(phi_le)
  vdot_fan/1 -> Verdunstung/4(Vdot_Fan)
  Qdot/1 -> Verdunstung/5(Qdot)
  t_ie/1 -> Verdunstung/6(t_ie)
  Strom/1(energy) -> energy/1

== system carnot/Source/Heat_Exchanger/Radiator_AIV/Troom ==
  "[AIV]" : Inport
  Sum4 : Sum  Inputs=1  SaturateOnIntegerOverflow=on  InputSameDT=on  OutDataTypeStr=Inherit: Same as first input
  gain : Gain  Gain=0.5  SaturateOnIntegerOverflow=on  OutDataTypeStr=Inherit: Same as input  ParamDataTypeStr=Inherit: Same as input
  select Tc Tr : Selector  InputPortWidth=9  IndexOptions=Index vector (dialog)  Indices=[2 3]  OutputSizes=1
  Troom : Outport
  wires:
  select Tc Tr/1 -> Sum4/1
  Sum4/1 -> gain/1
  gain/1 -> Troom/1  "Troom"
  "[AIV]"/1 -> select Tc Tr/1

== system carnot/Source/Heat_Pump/Ground_Source_Heat_Exchanger/Randbedingung 1 ==
  note: Qtot,i
  note: Qup,i
  note: Qdown,i
  T_Up : Inport
  T_Down : Inport  Port=2
  T_Earth(i,1) : Inport  Port=3
  Gain1 : Gain  Gain=L1/(2)  SaturateOnIntegerOverflow=on  OutDataTypeStr=Inherit: Same as input  ParamDataTypeStr=Inherit: Same as input
  Gain2 : Gain  Gain=L1/(2)  SaturateOnIntegerOverflow=on  OutDataTypeStr=Inherit: Same as input  ParamDataTypeStr=Inherit: Same as input
  Gain3 : Gain  Gain=(1)/L1  SaturateOnIntegerOverflow=on  OutDataTypeStr=Inherit: Same as input  ParamDataTypeStr=Inherit: Same as input
  Sum3 : Sum  Inputs=|-+  SaturateOnIntegerOverflow=on  InputSameDT=on  OutDataTypeStr=Inherit: Same as first input
  Sum4 : Sum  Inputs=-+  SaturateOnIntegerOverflow=on  InputSameDT=on  OutDataTypeStr=Inherit: Same as first input
  Sum5 : Sum  Inputs=|++  SaturateOnIntegerOverflow=on  InputSameDT=on  OutDataTypeStr=Inherit: Same as first input
  Sum6 : Sum  Inputs=|-+  SaturateOnIntegerOverflow=on  InputSameDT=on  OutDataTypeStr=Inherit: Same as first input
  T_Earth(i,0) : Outport
  wires:
  Sum6/1 -> T_Earth(i,0)/1
  T_Earth(i,1)/1 -> Sum6/2, Sum4/2, Sum3/2
  T_Up/1 -> Sum4/1
  T_Down/1 -> Sum3/1
  Gain3/1 -> Sum6/1
  Sum5/1 -> Gain3/1
  Gain2/1 -> Sum5/2
  Gain1/1 -> Sum5/1
  Sum4/1 -> Gain2/1
  Sum3/1 -> Gain1/1

== system carnot/Source/Heat_Pump/Ground_Source_Heat_Exchanger/Randbedingung 2 ==
  note: DeltaT
  note: T_Earth(i,DimRad)
  T_Earth(i,0) : Inport
  T_Earth(i,1) : Inport  Port=2
  Dd6 : Gain  Gain=c4  Multiplication=Matrix(K*u)  SaturateOnIntegerOverflow=on  OutDataTypeStr=Inherit: Same as input  ParamDataTypeStr=Inherit: Same as input
  Sum2 : Sum  Inputs=|+-  SaturateOnIntegerOverflow=on  InputSameDT=on  OutDataTypeStr=Inherit: Same as first input
  Sum3 : Sum  Inputs=+-  SaturateOnIntegerOverflow=on  InputSameDT=on  OutDataTypeStr=Inherit: Same as first input
  Tearth DimRad : Constant  Value=T_null  VectorParams1D=off
  g-function : Subsystem
  T_Earth(i,DimRad) Gew : Outport
  T_Earth(i,DimRad) : Outport  Port=2
  wires:
  g-function/1(DeltaT) -> Sum2/2
  Sum3/1 -> g-function/1(T(i,1)-T(i,0))
  Dd6/1 -> T_Earth(i,DimRad) Gew/1
  T_Earth(i,0)/1 -> Sum3/2
  T_Earth(i,1)/1 -> Sum3/1
  Tearth DimRad/1 -> Sum2/1
  Sum2/1 -> T_Earth(i,DimRad)/1, Dd6/1

== system carnot/Source/Heat_Pump/Ground_Source_Heat_Exchanger/Tdown ==
  In1 : Inport
  A mult : Product  Multiplication=Matrix(*)  RndMeth=Zero
  B mult : Product  Multiplication=Matrix(*)  RndMeth=Zero
  C mult : Product  Multiplication=Matrix(*)  RndMeth=Zero
  D mult : Product  Multiplication=Matrix(*)  RndMeth=Zero
  Integrator : Integrator  InitialCondition=Tdown_0
  Selector1 : Selector  InputPortWidth=DimAxi/2  IndexOptions=Index vector (dialog)  Indices=1  OutputSizes=1
  Selector2 : Selector  InputPortWidth=DimAxi/2  IndexOptions=Index vector (dialog)  Indices=2  OutputSizes=1
  Sum1 : Sum  Inputs=|++
  Sum2 : Sum  Inputs=++|
  Out1 : Outport
  Out2 : Outport  Port=2
  Out3 : Outport  Port=3
  wires:
  Sum2/1 -> Selector2/1, Selector1/1, Out1/1  "y"
  In1/1 -> B mult/2, D mult/2
  D mult/1 -> Sum2/1
  C mult/1 -> Sum2/2
  B mult/1 -> Sum1/1
  Sum1/1 -> Integrator/1  "Xdot"
  Integrator/1 -> A mult/2, C mult/2  "X"
  A mult/1 -> Sum1/2
  [B] -> B mult/1
  [A] -> A mult/1
  [C] -> C mult/1
  [D] -> D mult/1
  Selector1/1 -> Out2/1
  Selector2/1 -> Out3/1

== system carnot/Source/Heat_Pump/Ground_Source_Heat_Exchanger/Tup ==
  In1 : Inport
  A mult : Product  Multiplication=Matrix(*)  RndMeth=Zero
  B mult : Product  Multiplication=Matrix(*)  RndMeth=Zero
  C mult : Product  Multiplication=Matrix(*)  RndMeth=Zero
  D mult : Product  Multiplication=Matrix(*)  RndMeth=Zero
  Integrator : Integrator  InitialCondition=Tup_0
  Selector1 : Selector  InputPortWidth=DimAxi/2  IndexOptions=Index vector (dialog)  Indices=1  OutputSizes=1
  Selector2 : Selector  InputPortWidth=DimAxi/2  IndexOptions=Index vector (dialog)  Indices=2  OutputSizes=1
  Sum1 : Sum  Inputs=|++
  Sum2 : Sum  Inputs=++|
  Out1 : Outport
  Out2 : Outport  Port=2
  Out3 : Outport  Port=3
  wires:
  Sum2/1 -> Selector2/1, Selector1/1, Out1/1  "y"
  In1/1 -> B mult/2, D mult/2
  D mult/1 -> Sum2/1
  C mult/1 -> Sum2/2
  B mult/1 -> Sum1/1
  Sum1/1 -> Integrator/1  "Xdot"
  Integrator/1 -> A mult/2, C mult/2  "X"
  A mult/1 -> Sum1/2
  [Bu] -> B mult/1
  [Au] -> A mult/1
  [Cu] -> C mult/1
  [Du] -> D mult/1
  Selector1/1 -> Out2/1
  Selector2/1 -> Out3/1

== system carnot/Source/Heat_Pump/Ground_Source_Heat_Exchanger/mdot>0 ==
  In1 : Inport
  mdot : Inport  Port=2
  In4 : Inport  Port=3
  Add : Sum
  Fcn2 : Fcn  Expr=u>0
  Fcn3 : Fcn  Expr=u==0
  Product : Product  RndMeth=Zero
  Product1 : Product  RndMeth=Zero
  Out1 : Outport
  wires:
  Product/1 -> Add/1
  Product1/1 -> Add/2
  In1/1 -> Product/1
  Add/1 -> Out1/1
  In4/1 -> Product1/2
  mdot/1 -> Fcn2/1, Fcn3/1
  Fcn2/1 -> Product/2
  Fcn3/1 -> Product1/1

== system carnot/Source/Heat_Pump/Ground_Source_Heat_Exchanger/mdot>1 ==
  In1 : Inport
  mdot : Inport  Port=2
  In4 : Inport  Port=3
  Add : Sum
  Fcn2 : Fcn  Expr=u>0
  Fcn3 : Fcn  Expr=u==0
  Product : Product  RndMeth=Zero
  Product1 : Product  RndMeth=Zero
  Out1 : Outport
  wires:
  Product/1 -> Add/1
  Product1/1 -> Add/2
  In1/1 -> Product/1
  Add/1 -> Out1/1
  In4/1 -> Product1/2
  mdot/1 -> Fcn2/1, Fcn3/1
  Fcn2/1 -> Product/2
  Fcn3/1 -> Product1/1

== system carnot/Source/Heat_Pump/Ground_Source_Heat_Exchanger/mdot>2 ==
  In1 : Inport
  mdot : Inport  Port=2
  In4 : Inport  Port=3
  Add : Sum
  Fcn2 : Fcn  Expr=u>0
  Fcn3 : Fcn  Expr=u==0
  Product : Product  RndMeth=Zero
  Product1 : Product  RndMeth=Zero
  Out1 : Outport
  wires:
  Product/1 -> Add/1
  Product1/1 -> Add/2
  In1/1 -> Product/1
  Add/1 -> Out1/1
  In4/1 -> Product1/2
  mdot/1 -> Fcn2/1, Fcn3/1
  Fcn2/1 -> Product/2
  Fcn3/1 -> Product1/1

== system carnot/Source/Heat_Pump/Ground_Source_Heat_Exchanger/mdot>3 ==
  In1 : Inport
  mdot : Inport  Port=2
  In4 : Inport  Port=3
  Add : Sum
  Fcn2 : Fcn  Expr=u>0
  Fcn3 : Fcn  Expr=u==0
  Product : Product  RndMeth=Zero
  Product1 : Product  RndMeth=Zero
  Out1 : Outport
  wires:
  Product/1 -> Add/1
  Product1/1 -> Add/2
  In1/1 -> Product/1
  Add/1 -> Out1/1
  In4/1 -> Product1/2
  mdot/1 -> Fcn2/1, Fcn3/1
  Fcn2/1 -> Product/2
  Fcn3/1 -> Product1/1

== system carnot/Source/Heat_Pump/Ground_Source_Heat_Exchanger/mdot>4 ==
  In1 : Inport
  mdot : Inport  Port=2
  In4 : Inport  Port=3
  Add : Sum
  Fcn2 : Fcn  Expr=u>0
  Fcn3 : Fcn  Expr=u==0
  Product : Product  RndMeth=Zero
  Product1 : Product  RndMeth=Zero
  Out1 : Outport
  wires:
  Product/1 -> Add/1
  Product1/1 -> Add/2
  In1/1 -> Product/1
  Add/1 -> Out1/1
  In4/1 -> Product1/2
  mdot/1 -> Fcn2/1, Fcn3/1
  Fcn2/1 -> Product/2
  Fcn3/1 -> Product1/1

== system carnot/Source/Heat_Pump/Ground_Source_Heat_Exchanger/mdot>5 ==
  In1 : Inport
  mdot : Inport  Port=2
  In4 : Inport  Port=3
  Add : Sum
  Fcn2 : Fcn  Expr=u>0
  Fcn3 : Fcn  Expr=u==0
  Product : Product  RndMeth=Zero
  Product1 : Product  RndMeth=Zero
  Out1 : Outport
  wires:
  Product/1 -> Add/1
  Product1/1 -> Add/2
  In1/1 -> Product/1
  Add/1 -> Out1/1
  In4/1 -> Product1/2
  mdot/1 -> Fcn2/1, Fcn3/1
  Fcn2/1 -> Product/2
  Fcn3/1 -> Product1/1

== system carnot/Source/Heat_Pump/Ground_Source_Heat_Exchanger/mdot>6 ==
  In1 : Inport
  mdot : Inport  Port=2
  In4 : Inport  Port=3
  Add : Sum
  Fcn2 : Fcn  Expr=u>0
  Fcn3 : Fcn  Expr=u==0
  Product : Product  RndMeth=Zero
  Product1 : Product  RndMeth=Zero
  Out1 : Outport
  wires:
  Product/1 -> Add/1
  Product1/1 -> Add/2
  In1/1 -> Product/1
  Add/1 -> Out1/1
  In4/1 -> Product1/2
  mdot/1 -> Fcn2/1, Fcn3/1
  Fcn2/1 -> Product/2
  Fcn3/1 -> Product1/1

== system carnot/Source/Heat_Pump/Ground_Source_Heat_Exchanger/mdot>7 ==
  In1 : Inport
  mdot : Inport  Port=2
  In4 : Inport  Port=3
  Add : Sum
  Fcn2 : Fcn  Expr=u>0
  Fcn3 : Fcn  Expr=u==0
  Product : Product  RndMeth=Zero
  Product1 : Product  RndMeth=Zero
  Out1 : Outport
  wires:
  Product/1 -> Add/1
  Product1/1 -> Add/2
  In1/1 -> Product/1
  Add/1 -> Out1/1
  In4/1 -> Product1/2
  mdot/1 -> Fcn2/1, Fcn3/1
  Fcn2/1 -> Product/2
  Fcn3/1 -> Product1/1

== system carnot/Source/Solar_Thermal/Collector_EN12975/create_dataC ==
  acol : Inport
  THBin : Inport  Port=2
  THBout : Inport  Port=3
  Qdot : Inport  Port=4
  Tmean : Inport  Port=5
  WDB : Inport  Port=6
  Bus Creator : BusCreator  Inputs=6
  data_c : Outport
  wires:
  acol/1 -> Bus Creator/1  "Acol"
  THBin/1 -> Bus Creator/2  "THBin"
  THBout/1 -> Bus Creator/3  "THBout"
  WDB/1 -> Bus Creator/6  "WDB_surface"
  Bus Creator/1 -> data_c/1
  Qdot/1 -> Bus Creator/4  "Qdot"
  Tmean/1 -> Bus Creator/5  "Tmean"

== system carnot/Source/Solar_Thermal/IncidenceAngleModifier/IAM_Table ==
  note: q_solar_absorbed = F'(TauAlfa) (Kdir Idir + Kdfu Idfu)
  WDB : Inport
  Bus Selector : BusSelector  OutputSignals=Solar_Radiation_direct_surface,Solar_Radiation_diffuse_surface,Incidence_Angle_sun
  F'(tau*alfa) : Gain  Gain=fta  SaturateOnIntegerOverflow=on  OutDataTypeStr=Inherit: Same as input  ParamDataTypeStr=Inherit: Same as input
  IAM dfu : Gain  Gain=Kd  SaturateOnIntegerOverflow=on  OutDataTypeStr=Inherit: Same as input  ParamDataTypeStr=Inherit: Same as input
  Kb : Lookup  InputValues=angle  Table=Kb  SaturateOnIntegerOverflow=on
  Product1 : Product  SaturateOnIntegerOverflow=on  InputSameDT=on  OutDataTypeStr=Inherit: Same as first input
  Sum1 : Sum  SaturateOnIntegerOverflow=on  InputSameDT=on  OutDataTypeStr=Inherit: Same as first input
  Sum3 : Sum  SaturateOnIntegerOverflow=on  InputSameDT=on  OutDataTypeStr=Inherit: Same as first input
  qsolar : Outport
  Iglb : Outport  Port=2
  wires:
  F'(tau*alfa)/1 -> qsolar/1
  Sum1/1 -> Iglb/1
  Sum3/1 -> F'(tau*alfa)/1
  Kb/1 -> Product1/2
  Bus Selector/3 -> Kb/1  "<Incidence_Angle_sun>"
  Bus Selector/2 -> IAM dfu/1, Sum1/2  "<Solar_Radiation_diffuse_surface>"
  Bus Selector/1 -> Product1/1, Sum1/1  "<Solar_Radiation_direct_surface>"
  IAM dfu/1 -> Sum3/1
  Product1/1 -> Sum3/2
  WDB/1 -> Bus Selector/1

== system carnot/Source/Solar_Thermal/IncidenceAngleModifier/IAM_Table_KbL_KbT ==
  note: q_solar_absorbed = F'(TauAlfa) (Kdir Idir + Kdfu Idfu)
  WDB : Inport
  Bus Selector : BusSelector  OutputSignals=Solar_Radiation_direct_surface,Solar_Radiation_diffuse_surface,Incidence_Angle_longitudinal,Incidence_Angle_transversal
  F'(tau*alfa) : Gain  Gain=fta  SaturateOnIntegerOverflow=on  OutDataTypeStr=Inherit: Same as input  ParamDataTypeStr=Inherit: Same as input
  IAM dfu : Gain  Gain=Kd  SaturateOnIntegerOverflow=on  OutDataTypeStr=Inherit: Same as input  ParamDataTypeStr=Inherit: Same as input
  KbL : Lookup  InputValues=kblangle  Table=KbL  SaturateOnIntegerOverflow=on
  KbT : Lookup  InputValues=kbtangle  Table=KbT  SaturateOnIntegerOverflow=on
  Product1 : Product  Inputs=3  SaturateOnIntegerOverflow=on  InputSameDT=on  OutDataTypeStr=Inherit: Same as first input
  Scope1 : Scope  NumInputPorts=2
      settings: YMin=-5~-5  YMax=5~5  SaveName=ScopeData2
  Sum1 : Sum  SaturateOnIntegerOverflow=on  InputSameDT=on  OutDataTypeStr=Inherit: Same as first input
  Sum3 : Sum  SaturateOnIntegerOverflow=on  InputSameDT=on  OutDataTypeStr=Inherit: Same as first input
  qsolar : Outport
  Iglb : Outport  Port=2
  wires:
  IAM dfu/1 -> Scope1/1, Sum3/1
  F'(tau*alfa)/1 -> qsolar/1
  Sum1/1 -> Iglb/1
  Sum3/1 -> F'(tau*alfa)/1
  KbT/1 -> Product1/3
  KbL/1 -> Product1/2
  Bus Selector/3 -> KbL/1  "<Incidence_Angle_longitudinal>"
  Bus Selector/4 -> KbT/1  "<Incidence_Angle_transversal>"
  Bus Selector/2 -> IAM dfu/1, Sum1/2  "<Solar_Radiation_diffuse_surface>"
  Bus Selector/1 -> Product1/1, Sum1/1  "<Solar_Radiation_direct_surface>"
  Product1/1 -> Scope1/2, Sum3/2
  WDB/1 -> Bus Selector/1

== system carnot/Source/Solar_Thermal/IncidenceAngleModifier/IAM_b0 ==
  note: teta < 60°: Kdir = 1 - b0 * (1/cos(teta) -1)
      | teta > 60°: Kdir = (1 - b0) * (1 - (teta-60)/30)
  note: q_solar_absorbed = F'(TauAlfa) (Kdir Idir + Kdfu Idfu)
  WDB : Inport
  Bias : Bias  Bias=-1
  Bias1 : Bias  Bias=1
  Bias2 : Bias  Bias=1
  Bias3 : Bias  Bias=-60
  Bias4 : Bias  Bias=1
  Bus Selector : BusSelector  OutputSignals=Incidence_Angle_sun,Solar_Radiation_direct_surface,Solar_Radiation_diffuse_surface
  Compare To Constant : simulink/Logic and Bit Operations/Compare To Constant  relop=>=  const=60  OutDataTypeStr=uint8
  Constant : Constant  Value=1-b0
  Degrees to Radians : simulink_extras/Transformations/Degrees to Radians
  F'(tau*alfa) : Gain  Gain=fta  SaturateOnIntegerOverflow=on  OutDataTypeStr=Inherit: Same as input  ParamDataTypeStr=Inherit: Same as input
  IAM Kdiffuse : Gain  Gain=Kd  SaturateOnIntegerOverflow=on  OutDataTypeStr=Inherit: Same as input  ParamDataTypeStr=Inherit: Same as input
  Math Function : Math  Operator=reciprocal  SaturateOnIntegerOverflow=on
  Multiport Switch : MultiPortSwitch  Inputs=2
  Product : Product  RndMeth=Zero
  Product1 : Product  RndMeth=Zero
  Saturation : Saturate  UpperLimit=inf  LowerLimit=0
  Sum : Sum  SaturateOnIntegerOverflow=on  InputSameDT=on  OutDataTypeStr=Inherit: Same as first input
  Sum1 : Sum  SaturateOnIntegerOverflow=on  InputSameDT=on  OutDataTypeStr=Inherit: Same as first input
  Trigonometric Function : Trigonometry  Operator=cos
  b0 : Gain  Gain=-b0  SaturateOnIntegerOverflow=on  OutDataTypeStr=Inherit: Same as input  ParamDataTypeStr=Inherit: Same as input
  b1 : Gain  Gain=-1/30  SaturateOnIntegerOverflow=on  OutDataTypeStr=Inherit: Same as input  ParamDataTypeStr=Inherit: Same as input
  qsolar : Outport
  Iglb : Outport  Port=2
  wires:
  Bias4/1 -> Product1/1
  Product1/1 -> Multiport Switch/3
  Constant/1 -> Product1/2
  b1/1 -> Bias4/1
  Bias3/1 -> b1/1
  Multiport Switch/1 -> Saturation/1
  Bias1/1 -> Multiport Switch/2
  Bias2/1 -> Multiport Switch/1
  Compare To Constant/1 -> Bias2/1
  Saturation/1 -> Product/1
  WDB/1 -> Bus Selector/1
  Bus Selector/3 -> IAM Kdiffuse/1, Sum1/2  "<Solar_Radiation_diffuse_surface>"
  Bus Selector/1 -> Degrees to Radians/1, Compare To Constant/1, Bias3/1  "<Incidence_Angle_sun>"
  Bus Selector/2 -> Product/2, Sum1/1  "<Solar_Radiation_direct_surface>"
  IAM Kdiffuse/1 -> Sum/2
  Product/1 -> Sum/1
  Sum/1 -> F'(tau*alfa)/1
  F'(tau*alfa)/1 -> qsolar/1
  Sum1/1 -> Iglb/1
  Degrees to Radians/1 -> Trigonometric Function/1
  Trigonometric Function/1 -> Math Function/1
  Math Function/1 -> Bias/1
  Bias/1 -> b0/1
  b0/1 -> Bias1/1

== system carnot/Source/Solar_Thermal/IncidenceAngleModifier/Theoretical_Collector_Optics ==
  WDB : Inport
  IAM_Table : carnot/Source/Solar_Thermal/IncidenceAngleModifier/IAM_Table  fta=FTA  angle=teta  Kb=kb  Kd=kd
  qsolar : Outport
  Iglb : Outport  Port=2
  wires:
  WDB/1 -> IAM_Table/1
  IAM_Table/1 -> qsolar/1
  IAM_Table/2 -> Iglb/1

== system carnot/Source/Solar_Thermal/PressureDropCollector/pressure_drop_calculated_for_header_riser_water ==
  T : Inport
  mdot : Inport  Port=2
  p : Inport  Port=3
  lin_qua : Inport  Port=4
  1/acol : Gain  Gain=1/acol  SaturateOnIntegerOverflow=on  OutDataTypeStr=Inherit: Same as input  ParamDataTypeStr=Inherit: Same as input
  Aonecol : Gain  Gain=aonecol  SaturateOnIntegerOverflow=on  OutDataTypeStr=Inherit: Same as input  ParamDataTypeStr=Inherit: Same as input
  Demux3 : Demux  Outputs=2
  Look-Up Table (2-D) : Lookup2D  RowIndex=0:50:200  ColumnIndex=0:0.01:0.05  Table="[0 121.8750 261.8368 419.7212 595.443 788.9438; 0 44.3145 106.6853 186.9531 285.0355 400.8755; 0 29.8974 78.2964 145.0362 230.0334 333.2306; 0 24.2577 67.8077 130.4839 212.2001 312.8971; 0  21.7174 64.2104 127.3018 210.8995 314.9402]"  SaturateOnIntegerOverflow=on  InputSameDT=on
  Math Function : Math  Operator=square  SaturateOnIntegerOverflow=on
  Mux : Mux  Inputs=2
  Product : Product  Inputs=*/  SaturateOnIntegerOverflow=on  InputSameDT=on  OutDataTypeStr=Inherit: Same as first input
  Sum : Sum  Inputs=-+  SaturateOnIntegerOverflow=on  InputSameDT=on  OutDataTypeStr=Inherit: Same as first input
  Sum1 : Sum  SaturateOnIntegerOverflow=on  InputSameDT=on  OutDataTypeStr=Inherit: Same as first input
  p_out : Outport
  lq_out : Outport  Port=2
  wires:
  Look-Up Table (2-D)/1 -> Aonecol/1
  T/1 -> Look-Up Table (2-D)/1
  1/acol/1 -> Look-Up Table (2-D)/2
  mdot/1 -> 1/acol/1, Math Function/1
  lin_qua/1 -> Demux3/1
  Demux3/2 -> Sum1/2
  Sum1/1 -> Product/1
  Math Function/1 -> Product/2
  Product/1 -> Mux/2
  Mux/1 -> lq_out/1
  Demux3/1 -> Mux/1
  Sum/1 -> p_out/1
  p/1 -> Sum/2
  Aonecol/1 -> Sum/1, Sum1/1

== system carnot/Source/Solar_Thermal/PressureDropCollector/pressure_drop_for_measured_data_water ==
  T : Inport
  mdot : Inport  Port=2
  p : Inport  Port=3
  lin_qua : Inport  Port=4
  1/Ttest : Gain  Gain=1/ttest  SaturateOnIntegerOverflow=on  OutDataTypeStr=Inherit: Same as input  ParamDataTypeStr=Inherit: Same as input
  Aonecol/ (Acol*mdottest) : Gain  Gain=aonecol/(acol*mdottest)  SaturateOnIntegerOverflow=on  OutDataTypeStr=Inherit: Same as input  ParamDataTypeStr=Inherit: Same as input
  Demux3 : Demux  Outputs=2
  Look-Up Table (2-D) : Lookup2D  RowIndex=0:2.5:10  ColumnIndex=0:0.6175:3.0875  Table="pdroptest*[0  0.7699  1.6541  2.6516  3.7617  4.9841;  0  0.28  0.674  1.1811  1.8007  2.5325;  0  0.1889  0.4946  0.9163  1.4532  2.1052;  0  0.1532  0.4284  0.8243  1.3406  1.9767;  0  0.1372  0.4056  0.8042  1.3323  1.9896]"  SaturateOnIntegerOverflow=on  InputSameDT=on
  Math Function : Math  Operator=square  SaturateOnIntegerOverflow=on
  Mux : Mux  Inputs=2
  Product : Product  Inputs=*/  SaturateOnIntegerOverflow=on  InputSameDT=on  OutDataTypeStr=Inherit: Same as first input
  Sum : Sum  Inputs=-+  SaturateOnIntegerOverflow=on  InputSameDT=on  OutDataTypeStr=Inherit: Same as first input
  Sum1 : Sum  SaturateOnIntegerOverflow=on  InputSameDT=on  OutDataTypeStr=Inherit: Same as first input
  p_out : Outport
  lq_out : Outport  Port=2
  wires:
  Aonecol/ (Acol*mdottest)/1 -> Look-Up Table (2-D)/2
  1/Ttest/1 -> Look-Up Table (2-D)/1
  T/1 -> 1/Ttest/1
  lin_qua/1 -> Demux3/1
  Demux3/2 -> Sum1/2
  Sum1/1 -> Product/1
  Math Function/1 -> Product/2
  Product/1 -> Mux/2
  Mux/1 -> lq_out/1
  Demux3/1 -> Mux/1
  Sum/1 -> p_out/1
  p/1 -> Sum/2
  Look-Up Table (2-D)/1 -> Sum/1, Sum1/1
  mdot/1 -> Aonecol/ (Acol*mdottest)/1, Math Function/1

== system carnot/Source/Solar_Thermal/PressureDropCollector/pressure_drop_quadratic_fitted_data ==
  T : Inport
  mdot : Inport  Port=2
  p : Inport  Port=3
  lin_qua : Inport  Port=4
  Aonecol/Acol : Gain  Gain=aonecol/acol  SaturateOnIntegerOverflow=on  OutDataTypeStr=Inherit: Same as input  ParamDataTypeStr=Inherit: Same as input
  Demux3 : Demux  Outputs=2
  Mux : Mux  Inputs=2
  Sum : Sum  Inputs=-+  SaturateOnIntegerOverflow=on  InputSameDT=on  OutDataTypeStr=Inherit: Same as first input
  Sum1 : Sum  SaturateOnIntegerOverflow=on  InputSameDT=on  OutDataTypeStr=Inherit: Same as first input
  Sum2 : Sum  SaturateOnIntegerOverflow=on  InputSameDT=on  OutDataTypeStr=Inherit: Same as first input
  T-correction : Lookup  InputValues=[0 400]  Table=[1 1]  SaturateOnIntegerOverflow=on
  const : Constant  Value=b
  const1 : Constant  Value=a
  dp per collector : DotProduct  OutDataTypeStr=Inherit: Inherit via internal rule
  pressuredrop : Fcn  Expr=(a*u[1]+b)*u[1]
  p_out : Outport
  lq_out : Outport  Port=2
  wires:
  mdot/1 -> Aonecol/Acol/1
  Aonecol/Acol/1 -> pressuredrop/1
  T/1 -> T-correction/1
  Sum2/1 -> Mux/1
  const1/1 -> Sum1/1
  const/1 -> Sum2/1
  Demux3/1 -> Sum2/2
  Sum1/1 -> Mux/2
  Sum/1 -> p_out/1
  dp per collector/1 -> Sum/1
  p/1 -> Sum/2
  Mux/1 -> lq_out/1
  Demux3/2 -> Sum1/2
  lin_qua/1 -> Demux3/1
  T-correction/1 -> dp per collector/1
  pressuredrop/1 -> dp per collector/2

== system carnot/Source/Solar_Thermal/PressureDropCollector/pressure_drop_quadratic_fitted_data_water ==
  T : Inport
  mdot : Inport  Port=2
  p : Inport  Port=3
  lin_qua : Inport  Port=4
  Aonecol/Acol : Gain  Gain=aonecol/acol  SaturateOnIntegerOverflow=on  OutDataTypeStr=Inherit: Same as input  ParamDataTypeStr=Inherit: Same as input
  Demux3 : Demux  Outputs=2
  Mux : Mux  Inputs=2
  Sum : Sum  Inputs=-+  SaturateOnIntegerOverflow=on  InputSameDT=on  OutDataTypeStr=Inherit: Same as first input
  Sum1 : Sum  SaturateOnIntegerOverflow=on  InputSameDT=on  OutDataTypeStr=Inherit: Same as first input
  Sum2 : Sum  SaturateOnIntegerOverflow=on  InputSameDT=on  OutDataTypeStr=Inherit: Same as first input
  T-correction fluid Water : Lookup  InputValues=0:20:200  Table="[0.9985  1.0  1.006  1.0154  1.0275  1.0419  1.0590  1.0794  1.1045  1.1367  1.1795]"  SaturateOnIntegerOverflow=on
  const : Constant  Value=b
  const1 : Constant  Value=a
  dp per collector : DotProduct  InputSameDT=on  OutDataTypeStr=Inherit: Inherit via internal rule
  pressuredrop : Fcn  Expr=(a*u[1]+b)*u[1]
  p_out : Outport
  lq_out : Outport  Port=2
  wires:
  pressuredrop/1 -> dp per collector/2
  T-correction fluid Water/1 -> dp per collector/1
  lin_qua/1 -> Demux3/1
  Demux3/2 -> Sum1/2
  Mux/1 -> lq_out/1
  p/1 -> Sum/2
  dp per collector/1 -> Sum/1
  Sum/1 -> p_out/1
  Sum1/1 -> Mux/2
  Demux3/1 -> Sum2/2
  const/1 -> Sum2/1
  const1/1 -> Sum1/1
  Sum2/1 -> Mux/1
  T/1 -> T-correction fluid Water/1
  Aonecol/Acol/1 -> pressuredrop/1
  mdot/1 -> Aonecol/Acol/1
